simulink model "sf_while"  (R2017b)
settings: Solver=FixedStepDiscrete  StartTime=0.0  StopTime=1  FixedStep=1  RelTol=1e-3  EnableMultiTasking=on
settings Model: FPTRunName=Active  ExtModeAutoUpdateStatusClock=off  Creator=The MathWorks, Inc.  LastModifiedBy=The MathWorks, Inc.
settings DataIOCC: LimitDataPoints=on  SaveFormat=Array  SignalLoggingName=sigsOut
settings OptimizationCC: ExpressionDepthLimit=2147483647  InitFltsAndDblsToZero=on  EfficientMapNaN2IntZero=off  LifeSpan=inf
settings DebuggingCC: SaveWithParameterizedLinksMsg=none  UnderspecifiedInitializationDetection=Classic  MergeDetectMultiDrivingBlocksExec=none  SignalResolutionControl=TryResolveAllWithWarning  MultiTaskDSMMsg=warning  MultiTaskCondExecSysMsg=none  FcnCallInpInsideContextMsg=warning  AllowSymbolicDim=off  StateNameClashWarn=warning  SFUnexpectedBacktrackingDiag=warning  SFNoUnconditionalDefaultTransitionDiag=warning  SFExecutionAtInitializationDiag=none
settings HardwareCC: ProdBitPerPointer=32  ProdBitPerSizeT=32  ProdBitPerPtrDiffT=32  ProdLargestAtomicFloat=None  ProdIntDivRoundTo=Undefined  ProdEndianess=Unspecified  ProdWordSize=32  ProdHWDeviceType=32-bit Generic  TargetUnknown=on
settings ModelReferenceCC: PropagateSignalLabelsOutOfModel=off
settings SFSimCC: SimParseCustomCode=off
settings CodeAppCC: StateflowObjectComments=on
settings GRTTargetCC: TargetFcnLib=ansi_tfl_tmw.mat  TargetLangStandard=C89/C90 (ANSI)  GeneratePreprocessorConditionals=Disable all  CombineOutputUpdateFcns=off  GRTInterface=on
settings ConfigComp: CovMetricSettings=dcmtr  CovHtmlReporting=on  CovSaveCumulativeToWorkspaceVar=on  CovSaveSingleToWorkspaceVar=on  CovExternalEMLEnable=off  CovSFcnEnable=off

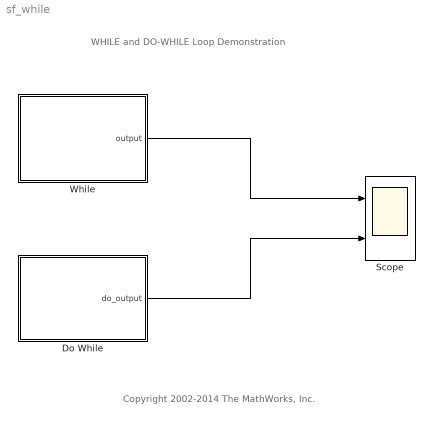
== system sf_while ==
  note: WHILE and DO-WHILE Loop Demonstration
  note: Copyright 2002-2014 The MathWorks, Inc.
  Do While : Stateflow chart  TreatAsAtomicUnit=on
  Scope : Scope  NumInputPorts=2
  While : Stateflow chart  TreatAsAtomicUnit=on
  wires:
  Do While/1(do_output) -> Scope/2
  While/1(output) -> Scope/1

== stateflow chart sf_while/While ==
  note: Equivalent C-Code:
      |
      | while(condition < 20)
      | {
      | while_output[i] = condition;
      | i++;
      | condition+=2;
      | }
  (default) -> (junction 17)
  (junction 17) -> (junction 14)
  (junction 14) -> (junction 16) [order 1] : [condition < 20]
  (junction 16) -> (junction 13) : {
      |   while_output[i] =condition;
      |   i++;
      |   condition+=2;
      | }
  (junction 13) -> (junction 14)
  (junction 14) -> (junction 15) [order 2] : {output=while_output;}
  data: condition local double; output output double size=[10 1]; i local double; while_output local double size=[10 1]

== stateflow chart sf_while/Do While ==
  note: Equivalent C-Code
      |
      | do {
      | do_output[i]=condition;
      | condition+=2;
      | i++;
      | } while(condition<20);
  (default) -> (junction 14)
  (junction 15) -> (junction 14)
  (junction 14) -> (junction 13) : {
      |   do_output[i]=condition;
      |   condition+=2;
      |   i++;
      | }
  (junction 13) -> (junction 15) [order 1] : [condition<20]
  (junction 13) -> (junction 12) [order 2]
  data: i local double; do_output output double size=[11 1]; condition local double
